simulink model "PI"  (R2020b)
settings: Solver=VariableStepAuto  StartTime=0.0  StopTime=10  RelTol=1e-3
values from neighbouring files (symbols this model uses):
  Ki = 35.0    [CC_data.sldd]
  Kp = 800.0    [CC_data.sldd]
settings Model: DataDictionary=CC_data.sldd  Creator=Varun  LastModifiedBy=Varun
settings DataIOCC: SaveOutput=off  SaveTime=off

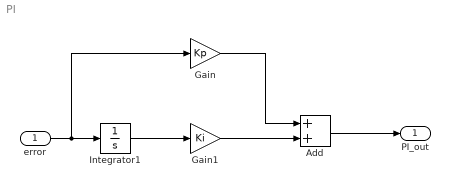
== system PI ==
  error : Inport  OutDataTypeStr=double  PortDimensions=1  SampleTime=0
  Add : Sum
  Gain : Gain  Gain=Kp
  Gain1 : Gain  Gain=Ki
  Integrator1 : Integrator
  PI_out : Outport  OutDataTypeStr=double  PortDimensions=1  SampleTime=0
  wires:
  Integrator1/1 -> Gain1/1
  Gain1/1 -> Add/2
  Gain/1 -> Add/1
  Add/1 -> PI_out/1
  error/1 -> Integrator1/1, Gain/1
